simulink model "untitled1"  (R2020b)
settings: Solver=VariableStepAuto  StartTime=0.0  StopTime=10.0  RelTol=1e-3
values from neighbouring files (symbols this model uses):
  th1 = 3.1    [lab2.m]
  th2 = 9.5    [lab2.m]
  th3 = 0.24    [lab2.m]
  th4 = 0.77    [lab2.m]
settings Model: Creator=ajankowi  LastModifiedBy=ajankowi

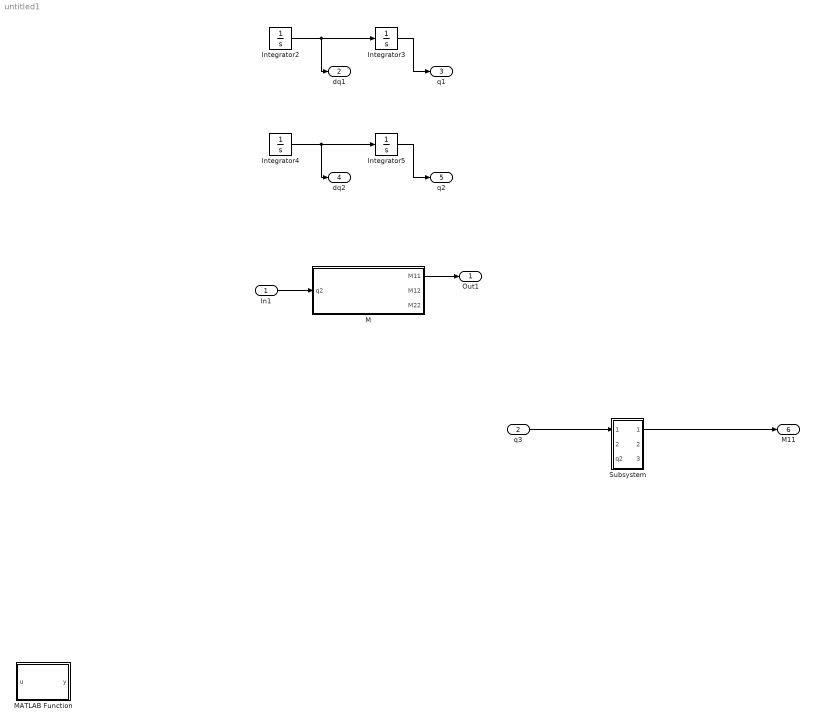
== system untitled1 ==
  In1 : Inport
  q3 : Inport  Port=2
  Integrator{2..5} (4 alike) : Integrator
  M : Subsystem
  MATLAB Function : MATLAB Function  TreatAsAtomicUnit=on
  Subsystem : Subsystem
  Out1 : Outport
  dq1 : Outport  Port=2
  q1 : Outport  Port=3
  dq2 : Outport  Port=4
  q2 : Outport  Port=5
  M11 : Outport  Port=6
  wires:
  In1/1 -> M/1(q2)
  M/1(M11) -> Out1/1
  Integrator5/1 -> q2/1
  Integrator4/1 -> dq2/1, Integrator5/1
  Integrator3/1 -> q1/1
  Integrator2/1 -> dq1/1, Integrator3/1
  q3/1 -> Subsystem/1(dq2)
  Subsystem/1(C11) -> M11/1

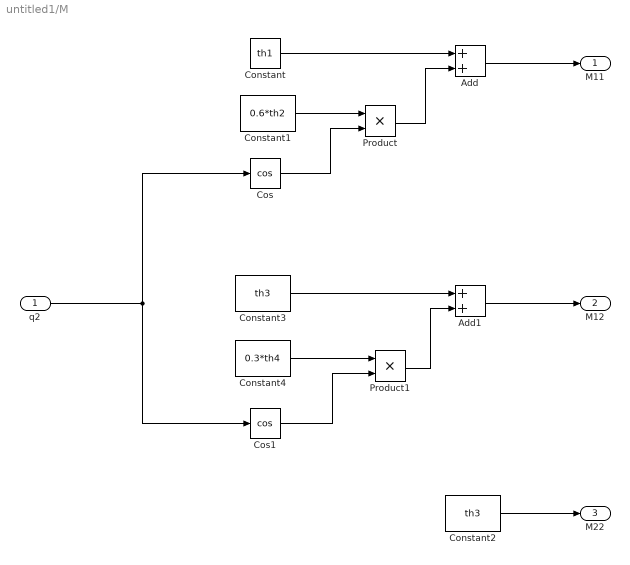
== system untitled1/M ==
  q2 : Inport
  Add : Sum
  Add1 : Sum
  Constant : Constant  Value=th1
  Constant1 : Constant  Value=0.6*th2
  Constant2 : Constant  Value=th3
  Constant3 : Constant  Value=th3
  Constant4 : Constant  Value=0.3*th4
  Cos : Trigonometry  Operator=cos
  Cos1 : Trigonometry  Operator=cos
  Product : Product
  Product1 : Product
  M11 : Outport
  M12 : Outport  Port=2
  M22 : Outport  Port=3
  wires:
  q2/1 -> Cos/1, Cos1/1
  Constant/1 -> Add/1
  Product/1 -> Add/2
  Constant1/1 -> Product/1
  Add/1 -> M11/1
  Cos/1 -> Product/2
  Constant2/1 -> M22/1
  Add1/1 -> M12/1
  Constant3/1 -> Add1/1
  Constant4/1 -> Product1/1
  Cos1/1 -> Product1/2
  Product1/1 -> Add1/2

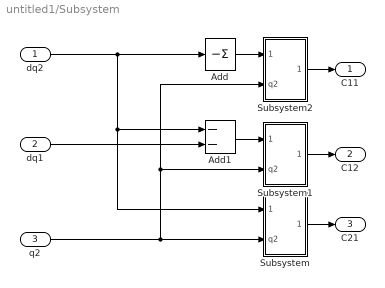
== system untitled1/Subsystem ==
  dq2 : Inport
  dq1 : Inport  Port=2
  q2 : Inport  Port=3
  Add : Sum  Inputs=-
  Add1 : Sum  Inputs=--
  Subsystem : Subsystem
  Subsystem1 : Subsystem
  Subsystem2 : Subsystem
  C11 : Outport
  C12 : Outport  Port=2
  C21 : Outport  Port=3
  wires:
  dq2/1 -> Subsystem/1(in1), Add1/1, Add/1
  dq1/1 -> Add1/2
  q2/1 -> Subsystem2/2(q2), Subsystem1/2(q2), Subsystem/2(q2)
  Subsystem/1(out2) -> C21/1
  Add1/1 -> Subsystem1/1(in1)
  Subsystem1/1(out2) -> C12/1
  Subsystem2/1(out2) -> C11/1
  Add/1 -> Subsystem2/1(in1)

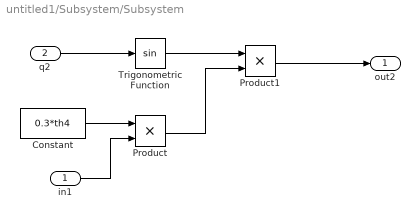
== system untitled1/Subsystem/Subsystem ==
  in1 : Inport
  q2 : Inport  Port=2
  Constant : Constant  Value=0.3*th4
  Product : Product
  Product1 : Product
  Trigonometric Function : Trigonometry
  out2 : Outport
  wires:
  Product1/1 -> out2/1
  in1/1 -> Product/2
  Trigonometric Function/1 -> Product1/1
  q2/1 -> Trigonometric Function/1
  Product/1 -> Product1/2
  Constant/1 -> Product/1

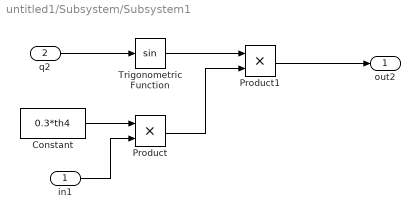
== system untitled1/Subsystem/Subsystem1 ==
  in1 : Inport
  q2 : Inport  Port=2
  Constant : Constant  Value=0.3*th4
  Product : Product
  Product1 : Product
  Trigonometric Function : Trigonometry
  out2 : Outport
  wires:
  Product1/1 -> out2/1
  in1/1 -> Product/2
  Trigonometric Function/1 -> Product1/1
  q2/1 -> Trigonometric Function/1
  Product/1 -> Product1/2
  Constant/1 -> Product/1

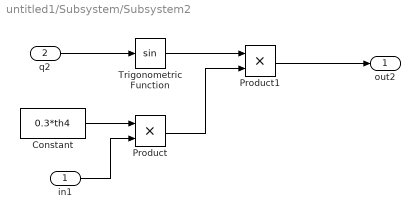
== system untitled1/Subsystem/Subsystem2 ==
  in1 : Inport
  q2 : Inport  Port=2
  Constant : Constant  Value=0.3*th4
  Product : Product
  Product1 : Product
  Trigonometric Function : Trigonometry
  out2 : Outport
  wires:
  Product1/1 -> out2/1
  in1/1 -> Product/2
  Trigonometric Function/1 -> Product1/1
  q2/1 -> Trigonometric Function/1
  Product/1 -> Product1/2
  Constant/1 -> Product/1

== matlab function untitled1/MATLAB Function ==
  data: u input; y output; data parameter
function y = fcn(u, data)

y = u;
